simulink model "Sim_project1"  (R2022b)
settings: Solver=ode45  StartTime=0.0  StopTime=sim_time  MaxStep=0.01  RelTol=1e-3
undefined symbols (not defined in the file): a, b, Cf, Cr, Iz, m, sine_amp, sine_freq, step_amp, U
settings Model: Creator=Forough  LastModifiedBy=Forough

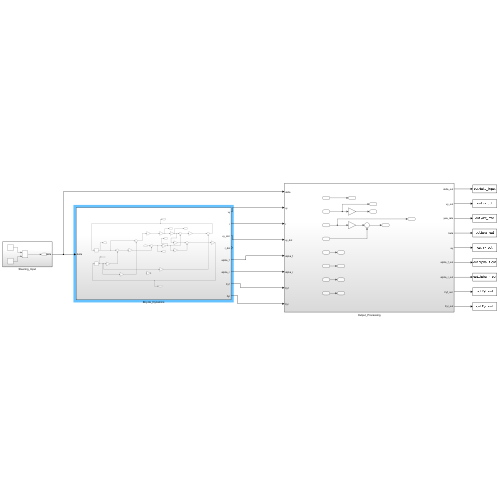
[thumbnail: Simulink's stored preview of the top-level diagram]
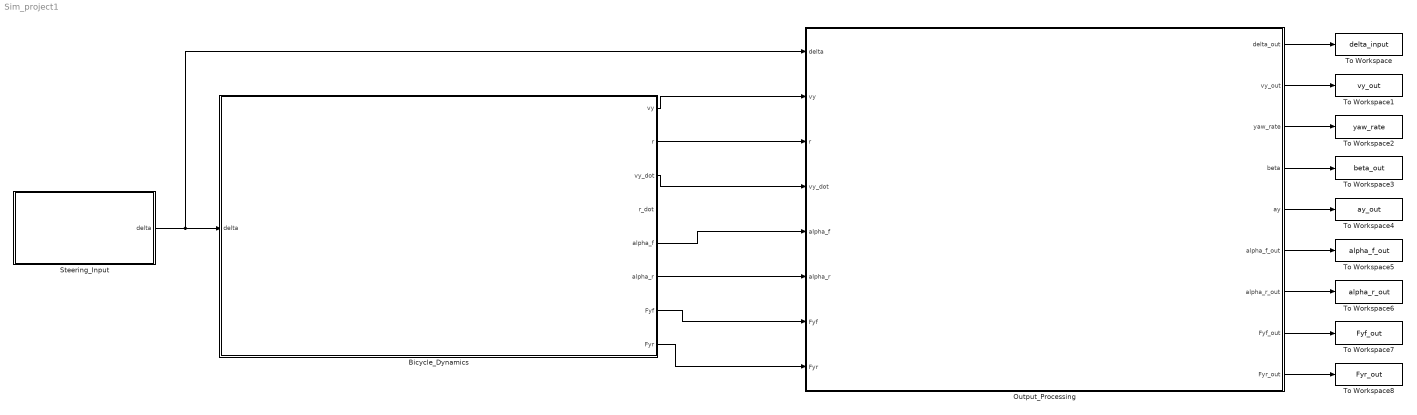
== system Sim_project1 ==
  Bicycle_Dynamics : Subsystem
  Output_Processing : Subsystem
  "Steering_Input " : Subsystem
  To Workspace : ToWorkspace  VariableName=delta_input  SaveFormat=Timeseries  SampleTime=-1
  To Workspace1 : ToWorkspace  VariableName=vy_out  SaveFormat=Timeseries  SampleTime=-1
  To Workspace2 : ToWorkspace  VariableName=yaw_rate  SaveFormat=Timeseries  SampleTime=-1
  To Workspace3 : ToWorkspace  VariableName=beta_out  SaveFormat=Timeseries  SampleTime=-1
  To Workspace4 : ToWorkspace  VariableName=ay_out  SaveFormat=Timeseries  SampleTime=-1
  To Workspace5 : ToWorkspace  VariableName=alpha_f_out  SaveFormat=Timeseries  SampleTime=-1
  To Workspace6 : ToWorkspace  VariableName=alpha_r_out  SaveFormat=Timeseries  SampleTime=-1
  To Workspace7 : ToWorkspace  VariableName=Fyf_out  SaveFormat=Timeseries  SampleTime=-1
  To Workspace8 : ToWorkspace  VariableName=Fyr_out  SaveFormat=Timeseries  SampleTime=-1
  wires:
  "Steering_Input "/1(delta) -> Output_Processing/1(delta), Bicycle_Dynamics/1(delta)
  Bicycle_Dynamics/1(vy) -> Output_Processing/2(vy)
  Bicycle_Dynamics/2(r) -> Output_Processing/3(r)
  Bicycle_Dynamics/3("vy_dot ") -> Output_Processing/4("vy_dot ")
  Bicycle_Dynamics/6("alpha_r ") -> Output_Processing/6("alpha_r ")
  Bicycle_Dynamics/5("alpha_f ") -> Output_Processing/5(alpha_f)
  Bicycle_Dynamics/7("Fyf ") -> Output_Processing/7("Fyf ")
  Bicycle_Dynamics/8(Fyr) -> Output_Processing/8(Fyr)
  Output_Processing/1(delta_out) -> To Workspace/1
  Output_Processing/2(vy_out) -> To Workspace1/1
  Output_Processing/3(yaw_rate) -> To Workspace2/1
  Output_Processing/4(beta) -> To Workspace3/1
  Output_Processing/5(ay) -> To Workspace4/1
  Output_Processing/6(alpha_f_out) -> To Workspace5/1
  Output_Processing/7(alpha_r_out) -> To Workspace6/1
  Output_Processing/8("Fyf_out ") -> To Workspace7/1
  Output_Processing/9(Fyr_out) -> To Workspace8/1

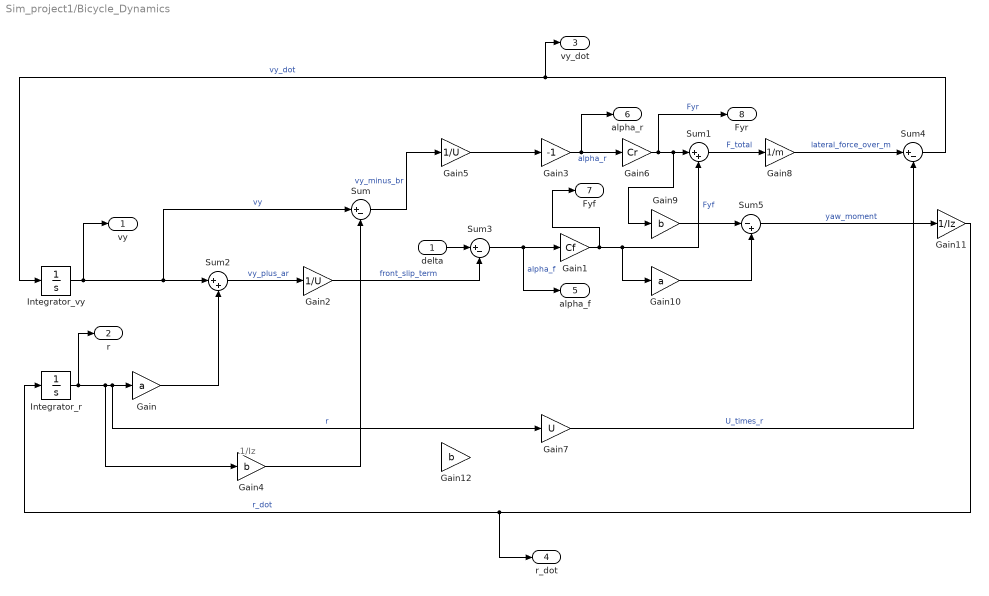
== system Sim_project1/Bicycle_Dynamics ==
  note: 1/Iz
  delta : Inport
  Gain : Gain  Gain=a
  Gain1 : Gain  Gain=Cf
  Gain10 : Gain  Gain=a
  Gain11 : Gain  Gain=1/Iz
  Gain12 : Gain  Gain=b
  Gain2 : Gain  Gain=1/U
  Gain3 : Gain  Gain=-1
  Gain4 : Gain  Gain=b
  Gain5 : Gain  Gain=1/U
  Gain6 : Gain  Gain=Cr
  Gain7 : Gain  Gain=U
  Gain8 : Gain  Gain=1/m
  Gain9 : Gain  Gain=b
  Integrator_r : Integrator
  Integrator_vy : Integrator
  Sum : Sum  Inputs=|+-
  Sum1 : Sum  Inputs=|++
  Sum2 : Sum  Inputs=|++
  Sum3 : Sum  Inputs=|+-
  Sum4 : Sum  Inputs=|+-
  Sum5 : Sum  Inputs=|-+
  vy : Outport
  r : Outport  Port=2
  "vy_dot " : Outport  Port=3
  r_dot : Outport  Port=4
  "alpha_f " : Outport  Port=5
  "alpha_r " : Outport  Port=6
  "Fyf " : Outport  Port=7
  Fyr : Outport  Port=8
  wires:
  Integrator_vy/1 -> vy/1, Sum/1, Sum2/1  "vy"
  Integrator_r/1 -> Gain4/1, Gain7/1, Gain/1, r/1  "r"
  Gain/1 -> Sum2/2
  Sum2/1 -> Gain2/1  "vy_plus_ar"
  Gain2/1 -> Sum3/2  "front_slip_term"
  Sum3/1 -> "alpha_f "/1, Gain1/1  "alpha_f"
  Gain1/1 -> "Fyf "/1, Gain10/1, Sum1/2  "Fyf"
  Gain4/1 -> Sum/2
  Sum/1 -> Gain5/1  "vy_minus_br"
  Gain5/1 -> Gain3/1
  Gain3/1 -> "alpha_r "/1, Gain6/1  "alpha_r"
  Gain6/1 -> Fyr/1, Gain9/1, Sum1/1  "Fyr"
  Sum1/1 -> Gain8/1  "F_total"
  Gain8/1 -> Sum4/1  "lateral_force_over_m"
  Gain7/1 -> Sum4/2  "U_times_r"
  Sum4/1 -> Integrator_vy/1, "vy_dot "/1  "vy_dot"
  Gain9/1 -> Sum5/1
  Gain10/1 -> Sum5/2
  Sum5/1 -> Gain11/1  "yaw_moment"
  Gain11/1 -> r_dot/1, Integrator_r/1  "r_dot"
  delta/1 -> Sum3/1

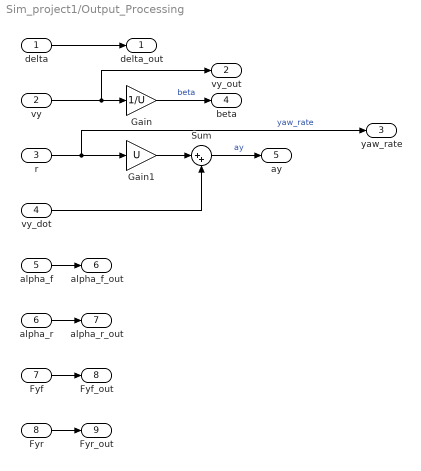
== system Sim_project1/Output_Processing ==
  delta : Inport
  vy : Inport  Port=2
  r : Inport  Port=3
  "vy_dot " : Inport  Port=4
  alpha_f : Inport  Port=5
  "alpha_r " : Inport  Port=6
  "Fyf " : Inport  Port=7
  Fyr : Inport  Port=8
  Gain : Gain  Gain=1/U
  Gain1 : Gain  Gain=U
  Sum : Sum  Inputs=|++
  delta_out : Outport
  vy_out : Outport  Port=2
  yaw_rate : Outport  Port=3
  beta : Outport  Port=4
  ay : Outport  Port=5
  alpha_f_out : Outport  Port=6
  alpha_r_out : Outport  Port=7
  "Fyf_out " : Outport  Port=8
  Fyr_out : Outport  Port=9
  wires:
  r/1 -> yaw_rate/1, Gain1/1  "yaw_rate"
  vy/1 -> vy_out/1, Gain/1
  Gain/1 -> beta/1  "beta"
  Gain1/1 -> Sum/1
  "vy_dot "/1 -> Sum/2
  Sum/1 -> ay/1  "ay"
  delta/1 -> delta_out/1
  alpha_f/1 -> alpha_f_out/1
  "alpha_r "/1 -> alpha_r_out/1
  "Fyf "/1 -> "Fyf_out "/1
  Fyr/1 -> Fyr_out/1

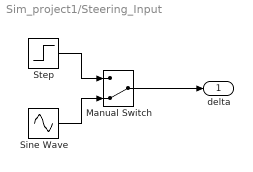
== system Sim_project1/Steering_Input  ==
  Manual Switch : ManualSwitch  CurrentSetting=0
  Sine Wave : Sin  Amplitude=sine_amp  Frequency=2*pi*sine_freq  SampleTime=0
  Step : Step  After=step_amp  SampleTime=0
  delta : Outport
  wires:
  Step/1 -> Manual Switch/1
  Sine Wave/1 -> Manual Switch/2
  Manual Switch/1 -> delta/1
